simulink model "lab03es1_sim"  (R2021b)
settings: Solver=FixedStepAuto  StartTime=0.0  StopTime=10000  FixedStep=0.1  RelTol=1e-3
values from neighbouring files (symbols this model uses):
  a = 1    [lab03es1.m]
settings Model: Creator=francescafornasier  LastModifiedBy=francescafornasier

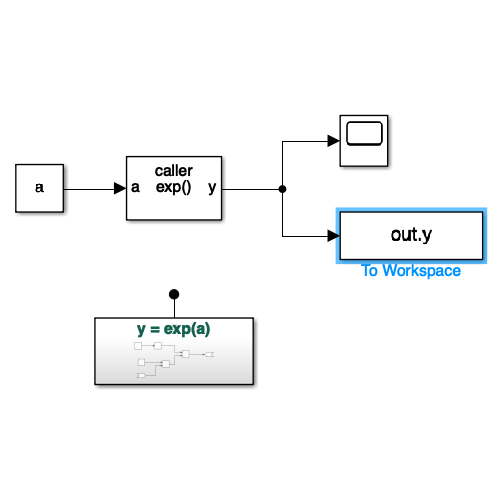
[thumbnail: Simulink's stored preview of the top-level diagram]
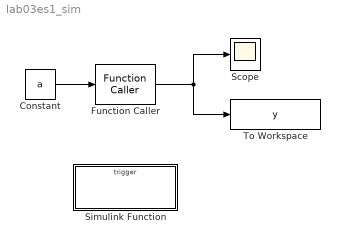
== system lab03es1_sim ==
  Constant : Constant  Value=a
  Function Caller : FunctionCaller  FunctionPrototype=y = exp(a)  InputArgumentSpecifications=<Enter example>  OutputArgumentSpecifications=<Enter example>
  Scope : Scope
  Simulink Function : Subsystem  TreatAsAtomicUnit=on
  To Workspace : ToWorkspace  VariableName=y  SaveFormat=Timeseries  SampleTime=-1
  wires:
  Function Caller/1 -> To Workspace/1, Scope/1
  Constant/1 -> Function Caller/1

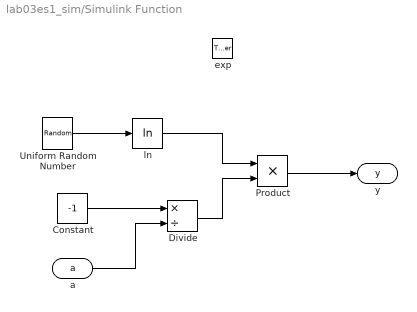
== system lab03es1_sim/Simulink Function ==
  exp : TriggerPort  TriggerType=function-call  IsSimulinkFunction=on  FunctionName=exp  FunctionVisibility=scoped  VariantControl=(inherit)
  Constant : Constant  Value=-1
  Divide : Product  Inputs=*/
  Product : Product
  Uniform Random Number : UniformRandomNumber  Minimum=0
  ln : Math  Operator=log  SaturateOnIntegerOverflow=on
  a : ArgIn  DisableCoverage=on  ArgumentName=a
  y : ArgOut  DisableCoverage=on  ArgumentName=y
  wires:
  a/1 -> Divide/2
  Constant/1 -> Divide/1
  Uniform Random Number/1 -> ln/1
  ln/1 -> Product/1
  Divide/1 -> Product/2
  Product/1 -> y/1
